simulink model "BuckyWagon_01"  (Simulink 7.7)
settings: Solver=FixedStepDiscrete  StartTime=0.0  StopTime=10.0  RelTol=1e-3
PreLoadFcn:
  | try, eval([bdroot '_setup']); catch, eval('model_setup', ''); end
InitFcn:
  | try, eval([bdroot '_setup']); catch, eval('model_setup', ''); end
undefined symbols (not defined in the file or in its folder): ECU565, High, Low, miniviewSetup, motohawk_build_version, motohawk_get_faults, motohawk_setup_toolchains, motohawk_trunc_name, motohawk_vardec_config_group, motohawk_vardec_path, tc, True
libraries: MotoHawk_lib x594, simulink x27, motohawk_control_primitives_lib x19, miniview_lib x10, MotoHawk_VDOGauge_lib x8, motohawk_engine_lib x5, motohawk_annotations_lib x1
(part 10 of 10)

== stateflow chart Foreground/Control Strategy/Calculations/kW calculation1/Downsapmle1 ==
  state Value_2
    du: count ++
    en: Val2 = Val_In
    count = 0
    state = 4
  state downsample_2
    du: count ++
    en:count = 0
    state = 3
  state Out
    en:state =5
    count = 0
    Out_1= Val1
    Out_2=Val2
    du: count++
  state downsample
    du:count++
    en: count = 0
    state = 1
  state Value_1
    du:count ++
    en: Val1 = Val_In
    count = 0
    state = 2
  Value_1 -> downsample_2 : [count >= 2]
  downsample -> Value_1 : [count >= numb_downsamp]
  downsample_2 -> Value_2 : [count >= numb_downsamp]
  (default) -> downsample
  Out -> downsample : [count >= 2]
  Value_2 -> Out : [count >=2]
  data: count local double; state local double; Out_1 output double; Out_2 output double; Val_In input double; numb_downsamp input double; Val1 local double; Val2 local double

== stateflow chart Foreground/Sensors/Eaton HV Charger/PluggedInDetect/Chart ==
  state Off
    entry:pluggedIn = 0;
  state countUp
    during:timer++;
  state CountDown
    during:timer--;
  state On
    entry:pluggedIn = 1;
  (default) -> Off
  Off -> countUp : [mainsOn]
  countUp -> CountDown [order 1] : [!mainsOn]
  CountDown -> countUp [order 2] : [mainsOn]
  CountDown -> Off [order 1] : [timer <= 0]
  On -> CountDown : [!mainsOn]
  countUp -> On [order 2] : [timer >= histTime]
  data: histTime input double; mainsOn input double; pluggedIn output boolean; timer local int16
